simulink model "HEX_Control_System"  (R2019b)
settings: Solver=ode45  StartTime=0.0  StopTime=10000  EnableMultiTasking=on
values from neighbouring files (symbols this model uses):
  K_l = 0.9    [HEX_Parameters.mat]
  T_l = 100    [HEX_Parameters.mat]
  v_h = u(1)    [HEX_Process.m]    (also in Projekt_feladatmegoldasok.m = (-(((K*S)/(ro_h*V_c*c_h))*(T_c-T_h))/(T_h_I-T_h))*V_h)
libraries: simulink x1
settings Model: Creator=martonl  LastModifiedBy=patti
settings DataIOCC: LimitDataPoints=on  SaveFormat=Array  ReturnWorkspaceOutputs=off
settings OptimizationCC: LifeSpan=inf
settings DebuggingCC: SFUnexpectedBacktrackingDiag=warning  SFNoUnconditionalDefaultTransitionDiag=warning  SFExecutionAtInitializationDiag=none  ArithmeticOperatorsInVariantConditions=warning
settings HardwareCC: ProdBitPerPointer=32  ProdBitPerSizeT=32  ProdBitPerPtrDiffT=32  ProdLargestAtomicFloat=None  ProdIntDivRoundTo=Undefined  ProdEndianess=Unspecified  ProdWordSize=32  ProdHWDeviceType=32-bit Generic
settings ModelReferenceCC: PropagateSignalLabelsOutOfModel=off
settings SFSimCC: SimUseLocalCustomCode=off  CustomCodeUndefinedFunction=UseInterfaceOnly
settings RTWCC: RTWUseLocalCustomCode=off
settings CodeAppCC: StateflowObjectComments=on
settings GRTTargetCC: TargetLangStandard=C89/C90 (ANSI)
settings ConfigComp: CovMetricSettings=dw  CovSaveCumulativeToWorkspaceVar=on  CovSaveSingleToWorkspaceVar=on  CovExternalEMLEnable=off  CovSFcnEnable=off

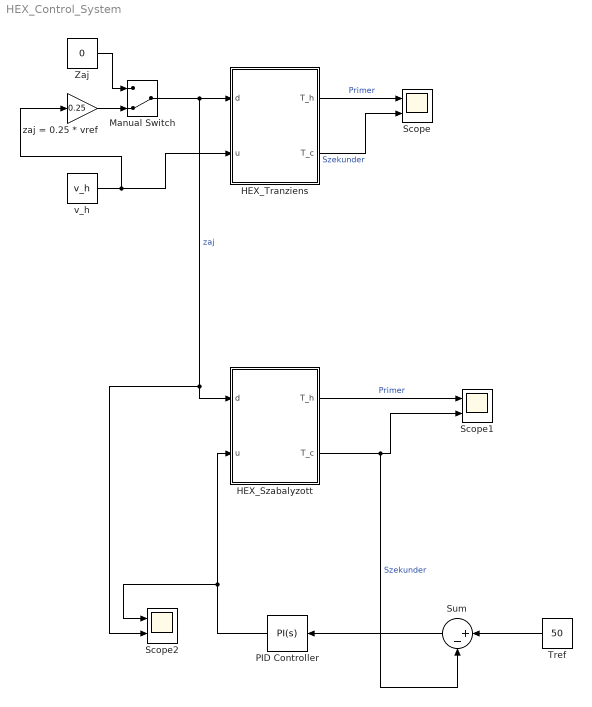
== system HEX_Control_System ==
  HEX_Szabalyzott : Subsystem
  HEX_Tranziens : Subsystem
  Manual Switch : ManualSwitch  CurrentSetting=0
  PID Controller : simulink/Continuous/PID Controller  Controller=PI  Form=Parallel  TimeDomain=Continuous-time  SampleTime=-1  IntegratorMethod=Forward Euler  FilterMethod=Forward Euler  ControllerParametersSource=internal  P=8.17612818539595e-06  I=1.40726232001797e-08  D=0  UseFilter=on  N=100  TunerSelectOption=Transfer Function Based (PID Tuner App)  InitialConditionSource=internal  InitialConditionForIntegrator=0  InitialConditionForFilter=0  DifferentiatorICPrevScaledInput=0  ExternalReset=none  TrackingMode=off  Kt=1  LimitOutput=off  UpperSaturationLimit=inf  LowerSaturationLimit=-inf  LinearizeAsGain=on  AntiWindupMode=none  Kb=1  POutMin=[]  POutMax=[]  IOutMin=[]  IOutMax=[]  DOutMin=[]  DOutMax=[]  NOutMin=[]  NOutMax=[]  SumOutMin=[]  SumOutMax=[]  SaturationOutMin=[]  SaturationOutMax=[]  PParamMin=[]  PParamMax=[]  IParamMin=[]  IParamMax=[]  DParamMin=[]  DParamMax=[]  NParamMin=[]  NParamMax=[]  KbParamMin=[]  KbParamMax=[]  KtParamMin=[]  KtParamMax=[]  KbOutMin=[]  KbOutMax=[]  KtOutMin=[]  KtOutMax=[]  IntegratorOutMin=[]  IntegratorOutMax=[]  FilterOutMin=[]  FilterOutMax=[]  SumI1OutMin=[]  SumI1OutMax=[]  SumI2OutMin=[]  SumI2OutMax=[]  SumI3OutMin=[]  SumI3OutMax=[]  SumI4OutMin=[]  SumI4OutMax=[]  SumDOutMin=[]  SumDOutMax=[]  DifferentiatorOutMin=[]  DifferentiatorOutMax=[]  FilterDiffOutCoefMin=[]  FilterDiffOutCoefMax=[]  ReciprocalOutMin=[]  ReciprocalOutMax=[]  SumDenOutMin=[]  SumDenOutMax=[]  SumNumOutMin=[]  SumNumOutMax=[]  DivideOutMin=[]  DivideOutMax=[]  IntegratorContinuousStateAttributes=''  IntegratorStateMustResolveToSignalObject=off  IntegratorRTWStateStorageClass=Auto  FilterContinuousStateAttributes=''  FilterStateMustResolveToSignalObject=off  FilterRTWStateStorageClass=Auto  ParallelPVariant=InternalParameters  IdealPVariant=Disabled  IVariant=InternalParameters  DVariant=Disabled  IntegratorVariant=Continuous  SatVariant=Disabled  AWVariant=Passthrough  PCopyVariant=Disabled  TRVariant=Disabled  FdbkBlocksVariant=Forward  IdealPFdbkVariant=Disabled  SatFdbkVariant=Disabled  DerivativeFilterVariant=Disabled  NVariant=Disabled  NCopyVariant=Disabled_SignalSpec  FilterICVariant=Disabled  IntegratorICVariant=InternalICs  ExternalResetVariant=Disabled  TRSumVariant=Passthrough  SumFdbkVariant=Disabled  SumVariant=Sum_PI
  Scope : Scope  NumInputPorts=2
  Scope1 : Scope  NumInputPorts=2
  Scope2 : Scope  NumInputPorts=2
  Sum : Sum  Inputs=|+-
  Tref : Constant  Value=50
  Zaj : Constant  Value=0
  v_h : Constant  Value=v_h
  zaj = 0.25 * vref : Gain  Gain=0.25
  wires:
  HEX_Tranziens/1(T_h) -> Scope/1  "Primer"
  HEX_Tranziens/2(T_c) -> Scope/2  "Szekunder"
  v_h/1 -> zaj = 0.25 * vref/1, HEX_Tranziens/2(u)
  Zaj/1 -> Manual Switch/1
  Manual Switch/1 -> Scope2/2, HEX_Szabalyzott/1(d), HEX_Tranziens/1(d)  "zaj"
  zaj = 0.25 * vref/1 -> Manual Switch/2
  HEX_Szabalyzott/2(T_c) -> Scope1/2, Sum/2  "Szekunder"
  HEX_Szabalyzott/1(T_h) -> Scope1/1  "Primer"
  Tref/1 -> Sum/1
  PID Controller/1 -> Scope2/1, HEX_Szabalyzott/2(u)
  Sum/1 -> PID Controller/1

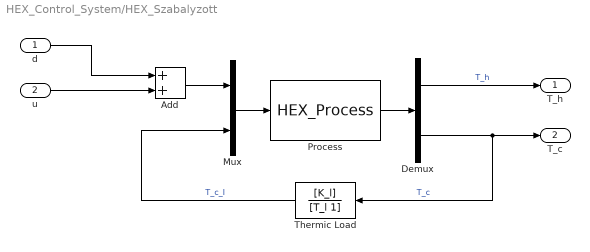
== system HEX_Control_System/HEX_Szabalyzott ==
  d : Inport
  u : Inport  Port=2
  Add : Sum
  Demux : Demux  Outputs=2
  Mux : Mux  Inputs=2
  Process : S-Function  FunctionName=HEX_Process  Parameters=process_parameters  SFunctionDeploymentMode=off  EnableBusSupport=off
  Thermic Load : TransferFcn  Numerator=[K_l]  Denominator=[T_l 1]
  T_h : Outport
  T_c : Outport  Port=2
  wires:
  Process/1 -> Demux/1
  Mux/1 -> Process/1
  Demux/2 -> T_c/1, Thermic Load/1  "T_c"
  Thermic Load/1 -> Mux/2  "T_c_I"
  Demux/1 -> T_h/1  "T_h"
  u/1 -> Add/2
  d/1 -> Add/1
  Add/1 -> Mux/1

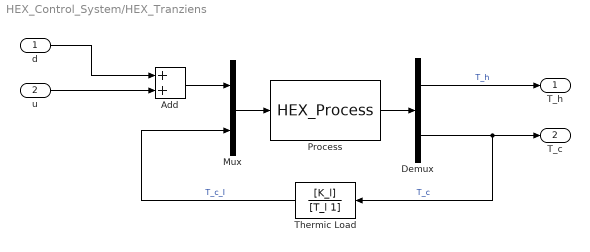
== system HEX_Control_System/HEX_Tranziens ==
  d : Inport
  u : Inport  Port=2
  Add : Sum
  Demux : Demux  Outputs=2
  Mux : Mux  Inputs=2
  Process : S-Function  FunctionName=HEX_Process  Parameters=process_parameters  SFunctionDeploymentMode=off  EnableBusSupport=off
  Thermic Load : TransferFcn  Numerator=[K_l]  Denominator=[T_l 1]
  T_h : Outport
  T_c : Outport  Port=2
  wires:
  Process/1 -> Demux/1
  Mux/1 -> Process/1
  Demux/2 -> T_c/1, Thermic Load/1  "T_c"
  Thermic Load/1 -> Mux/2  "T_c_I"
  Demux/1 -> T_h/1  "T_h"
  u/1 -> Add/2
  d/1 -> Add/1
  Add/1 -> Mux/1
